simulink model "PVTOL_FE_and_FTC_Sim"  (R2021a)
settings: Solver=VariableStepAuto  StartTime=0.0  StopTime=10  RelTol=1e-3
values from neighbouring files (symbols this model uses):
  A_brevebar = [A_breve E_breve;zeros(2,4) zeros(2,2)]    [Quadcopter_Fault_Parameters_and_Flags.m]
  B_brevebar = [B_breve;zeros(2,2)]    [Quadcopter_Fault_Parameters_and_Flags.m]
  Delta_p = [1 1;1 -1]    [Quadcopter_Fault_Parameters_and_Flags.m]
  Delta_q = [1 1 1 1;1 -1 -1 1;1 1 -1 -1;-1 1 -1 1]    [Quadcopter_Fault_Parameters_and_Flags.m]
  g = 9.8066    [Quadcopter_Fault_Parameters_and_Flags.m]
  g_bar = [g_bold;zeros(2,1)]    [Quadcopter_Fault_Parameters_and_Flags.m]
  Jx = 0.0022    [Quadcopter_Fault_Parameters_and_Flags.m]
  K_D_kesi = diag([0.08,0.08,0.22])    [Quadcopter_Fault_Parameters_and_Flags.m]
  K_D_omega = diag([0.2,0.2,0.5])    [Quadcopter_Fault_Parameters_and_Flags.m]
  K_P_kesi = diag([0.18,0.18,052])    [Quadcopter_Fault_Parameters_and_Flags.m]
  K_P_omega = diag([1.5,1.5,2])    [Quadcopter_Fault_Parameters_and_Flags.m]
  kesi_d = [0 0 0]'    [Quadcopter_Fault_Parameters_and_Flags.m]
  kesi_dot_d = [0 0 0]'    [Quadcopter_Fault_Parameters_and_Flags.m]
  l = 0.1785    [Quadcopter_Fault_Parameters_and_Flags.m]
  Lf1 = 50    [Quadcopter_Fault_Parameters_and_Flags.m]
  Lf2 = 50    [Quadcopter_Fault_Parameters_and_Flags.m]
  LPI_brevebar = (P^-1)*M    [Quadcopter_Fault_Parameters_and_Flags.m]
  Ly1 = 0.009    [Quadcopter_Fault_Parameters_and_Flags.m]
  Ly2 = 5    [Quadcopter_Fault_Parameters_and_Flags.m]
  m = 0.4080    (= 0.408)    [Quadcopter_Fault_Parameters_and_Flags.m]
  O_d = [0 0 0]'    [Quadcopter_Fault_Parameters_and_Flags.m]
  Omega_d = [0 0 0]'    [Quadcopter_Fault_Parameters_and_Flags.m]
  Phi_dot_init = 0    [Quadcopter_Fault_Parameters_and_Flags.m]
  Phi_init = 0    [Quadcopter_Fault_Parameters_and_Flags.m]
  y_dot_init = 0    [Quadcopter_Fault_Parameters_and_Flags.m]
  y_init = 0    [Quadcopter_Fault_Parameters_and_Flags.m]
  z_dot_init = 0    [Quadcopter_Fault_Parameters_and_Flags.m]
  z_init = 0    [Quadcopter_Fault_Parameters_and_Flags.m]
settings Model: PauseTimes=2  Creator=kiankhaneghahi  LastModifiedBy=kiankhaneghahi

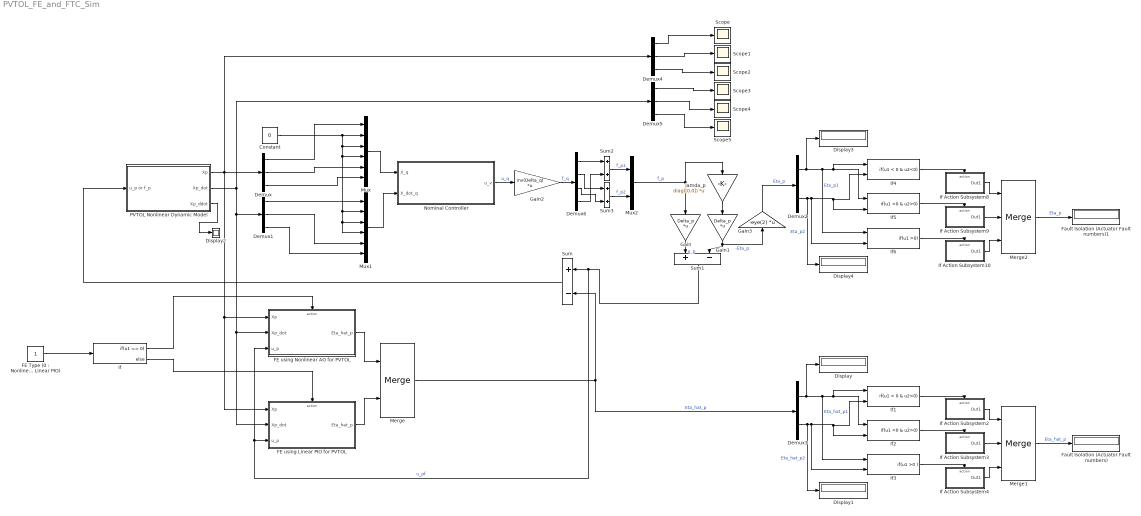
== system PVTOL_FE_and_FTC_Sim ==
  Constant : Constant  Value=0
  Demux{,1,4..5} (4 alike) : Demux  Outputs=3
  Demux2 : Demux  Outputs=2
  Demux3 : Demux  Outputs=2
  Demux6 : Demux
  Display{,1..4} (5 alike) : Display
  "FE Type (0 : Nonlinear AO - 1 : Linear PIO)" : Constant
  FE using Linear PIO for PVTOL : Subsystem
  FE using Nonlinear AO for PVTOL : Subsystem
  Fault Isolation (Actuator Fault numbers) : Display
  Fault Isolation (Actuator Fault numbers)1 : Display
  Gain : Gain  Gain=Delta_p  Multiplication=Matrix(K*u)
  Gain1 : Gain  Gain=Delta_p  Multiplication=Matrix(K*u)
  Gain2 : Gain  Gain=inv(Delta_q)  Multiplication=Matrix(K*u)
  Gain3 : Gain  Gain=-eye(2)  Multiplication=Matrix(K*u)
  If : If  IfExpression=u1 == 0
  If Action Subsystem10 : Subsystem  TreatAsAtomicUnit=on
  If Action Subsystem2 : Subsystem  TreatAsAtomicUnit=on
  If Action Subsystem3 : Subsystem  TreatAsAtomicUnit=on
  If Action Subsystem4 : Subsystem  TreatAsAtomicUnit=on
  If Action Subsystem8 : Subsystem  TreatAsAtomicUnit=on
  If Action Subsystem9 : Subsystem  TreatAsAtomicUnit=on
  If1 : If  NumInputs=2  IfExpression=u1 < 0 & u2<0  ShowElse=off
  If2 : If  NumInputs=2  IfExpression=u1 <0 & u2>0  ShowElse=off
  If3 : If  NumInputs=2  IfExpression=u1 >0  ShowElse=off
  If4 : If  NumInputs=2  IfExpression=u1 < 0 & u2<0  ShowElse=off
  If5 : If  NumInputs=2  IfExpression=u1 <0 & u2>0  ShowElse=off
  If6 : If  NumInputs=2  IfExpression=u1 >0  ShowElse=off
  Merge : Merge
  Merge1 : Merge  Inputs=3
  Merge2 : Merge  Inputs=3
  Mux : Mux  Inputs=6
  Mux1 : Mux  Inputs=6
  Mux2 : Mux  Inputs=2
  Nominal Controller : Subsystem
  PVTOL Nonlinear Dynamic Model : Subsystem
  Scope{,1..5} (6 alike) : Scope
  Sum : Sum  Inputs=+-
  Sum1 : Sum  Inputs=+-
  Sum2 : Sum
  Sum3 : Sum
  lamda_p : Gain  Gain=diag([0,0])  Multiplication=Matrix(K*u)
  wires:
  PVTOL Nonlinear Dynamic Model/1(Xp) -> Demux4/1, FE using Linear PIO for PVTOL/1(Xp), FE using Nonlinear AO for PVTOL/1(Xp), Demux/1
  PVTOL Nonlinear Dynamic Model/2(Xp_dot) -> Demux5/1, FE using Linear PIO for PVTOL/2(Xp_dot), FE using Nonlinear AO for PVTOL/2(Xp_dot), Demux1/1
  Mux/1 -> Nominal Controller/1(X_q)
  Demux/1 -> Mux/1
  Demux/2 -> Mux/5
  Demux/3 -> Mux/6
  Mux1/1 -> Nominal Controller/2(X_dot_q)
  Demux1/1 -> Mux1/1
  Demux1/2 -> Mux1/5
  Demux1/3 -> Mux1/6
  Constant/1 -> Mux1/4, Mux1/3, Mux1/2, Mux/4, Mux/3, Mux/2
  "FE Type (0 : Nonlinear AO - 1 : Linear PIO)"/1 -> If/1
  If/1 -> FE using Nonlinear AO for PVTOL/Action
  If/2 -> FE using Linear PIO for PVTOL/Action
  FE using Nonlinear AO for PVTOL/1(Eta_hat_p) -> Merge/1
  FE using Linear PIO for PVTOL/1(Eta_hat_p) -> Merge/2
  Sum1/1 -> FE using Linear PIO for PVTOL/3(u_p), FE using Nonlinear AO for PVTOL/3(u_p), Sum/1  "u_pf"
  Merge/1 -> Demux3/1, Sum/2  "Eta_hat_p"
  Sum/1 -> PVTOL Nonlinear Dynamic Model/1(u_p or f_p)
  If Action Subsystem4/1(Out1) -> Merge1/3
  Merge1/1 -> Fault Isolation (Actuator Fault numbers)/1  "Eta_hat_p"
  If1/1 -> If Action Subsystem2/Action
  Demux3/1 -> Display/1, If3/1, If1/1, If2/1  "Eta_hat_p1"
  If Action Subsystem3/1(Out1) -> Merge1/2
  Demux3/2 -> Display1/1, If3/2, If1/2, If2/2  "Eta_hat_p2"
  If Action Subsystem2/1(Out1) -> Merge1/1
  If3/1 -> If Action Subsystem4/Action
  If2/1 -> If Action Subsystem3/Action
  PVTOL Nonlinear Dynamic Model/3(Xp_ddot) -> Display2/1
  Demux4/1 -> Scope/1
  Demux4/2 -> Scope1/1
  Demux4/3 -> Scope2/1
  Demux5/1 -> Scope3/1
  Demux5/2 -> Scope4/1
  Demux5/3 -> Scope5/1
  Gain2/1 -> Demux6/1  "f_q"
  Gain/1 -> Sum1/1  "u_p"
  Gain1/1 -> Sum1/2, Gain3/1  "-Eta_p"
  lamda_p/1 -> Gain1/1
  Nominal Controller/1(u_v) -> Gain2/1  "u_q"
  Demux6/1 -> Sum2/1
  Demux6/4 -> Sum2/2
  Demux6/2 -> Sum3/1
  Demux6/3 -> Sum3/2
  Sum2/1 -> Mux2/1  "f_p1"
  Sum3/1 -> Mux2/2  "f_p2"
  Mux2/1 -> Gain/1, lamda_p/1  "f_p"
  Gain3/1 -> Demux2/1  "Eta_p"
  Merge2/1 -> Fault Isolation (Actuator Fault numbers)1/1  "Eta_p"
  Demux2/1 -> Display3/1, If6/1, If4/1, If5/1  "Eta_p1"
  If6/1 -> If Action Subsystem10/Action
  If4/1 -> If Action Subsystem8/Action
  If5/1 -> If Action Subsystem9/Action
  Demux2/2 -> Display4/1, If6/2, If4/2, If5/2  "Eta_p2"
  If Action Subsystem8/1(Out1) -> Merge2/1
  If Action Subsystem9/1(Out1) -> Merge2/2
  If Action Subsystem10/1(Out1) -> Merge2/3

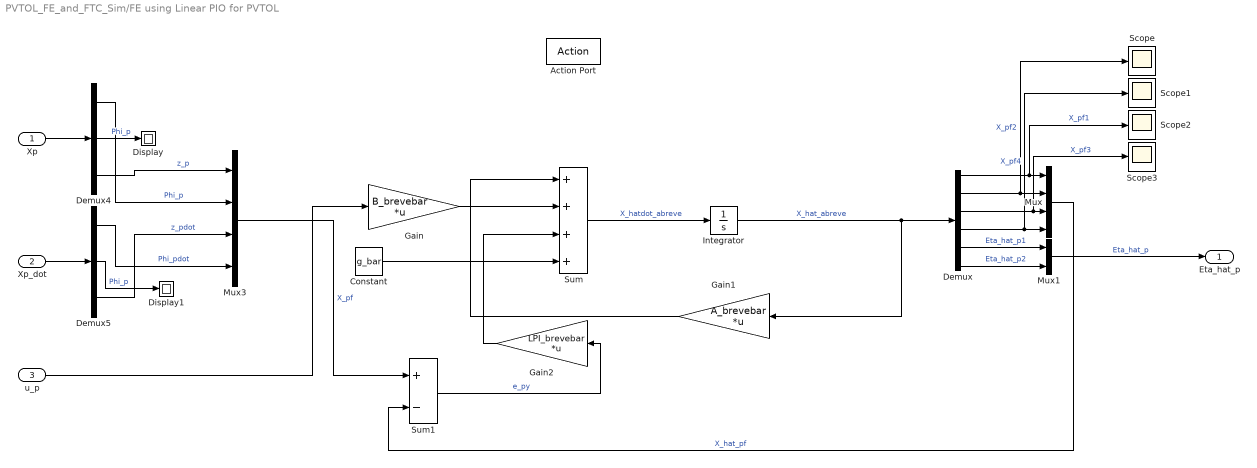
== system PVTOL_FE_and_FTC_Sim/FE using Linear PIO for PVTOL ==
  Xp : Inport
  Xp_dot : Inport  Port=2
  u_p : Inport  Port=3
  Action Port : ActionPort  ActionPortLabel=else
  Constant : Constant  Value=g_bar
  Demux : Demux  Outputs=6
  Demux4 : Demux  Outputs=3
  Demux5 : Demux  Outputs=3
  Display : Display
  Display1 : Display
  Gain : Gain  Gain=B_brevebar  Multiplication=Matrix(K*u)
  Gain1 : Gain  Gain=A_brevebar  Multiplication=Matrix(K*u)
  Gain2 : Gain  Gain=LPI_brevebar  Multiplication=Matrix(K*u)
  Integrator : Integrator
  Mux : Mux
  Mux1 : Mux  Inputs=2
  Mux3 : Mux
  Scope{,1..3} (4 alike) : Scope
  Sum : Sum  Inputs=++++
  Sum1 : Sum  Inputs=+-
  Eta_hat_p : Outport
  wires:
  Demux5/1 -> Mux3/4  "Phi_pdot"
  Xp/1 -> Demux4/1
  u_p/1 -> Gain/1
  Demux4/1 -> Mux3/2  "Phi_p"
  Demux4/3 -> Mux3/1  "z_p"
  Demux5/3 -> Mux3/3  "z_pdot"
  Xp_dot/1 -> Demux5/1
  Mux1/1 -> Eta_hat_p/1  "Eta_hat_p"
  Integrator/1 -> Demux/1, Gain1/1  "X_hat_abreve"
  Sum/1 -> Integrator/1  "X_hatdot_abreve"
  Gain1/1 -> Sum/1
  Gain/1 -> Sum/2
  Constant/1 -> Sum/4
  Demux/6 -> Mux1/2  "Eta_hat_p2"
  Demux/5 -> Mux1/1  "Eta_hat_p1"
  Mux/1 -> Sum1/2  "X_hat_pf"
  Demux4/2 -> Display/1  "Phi_p"
  Demux5/2 -> Display1/1  "Phi_p"
  Mux3/1 -> Sum1/1  "X_pf"
  Gain2/1 -> Sum/3
  Sum1/1 -> Gain2/1  "e_py"
  Demux/2 -> Scope/1, Mux/2  "X_pf2"
  Demux/3 -> Scope3/1, Mux/3  "X_pf3"
  Demux/1 -> Scope2/1, Mux/1  "X_pf1"
  Demux/4 -> Scope1/1, Mux/4  "X_pf4"

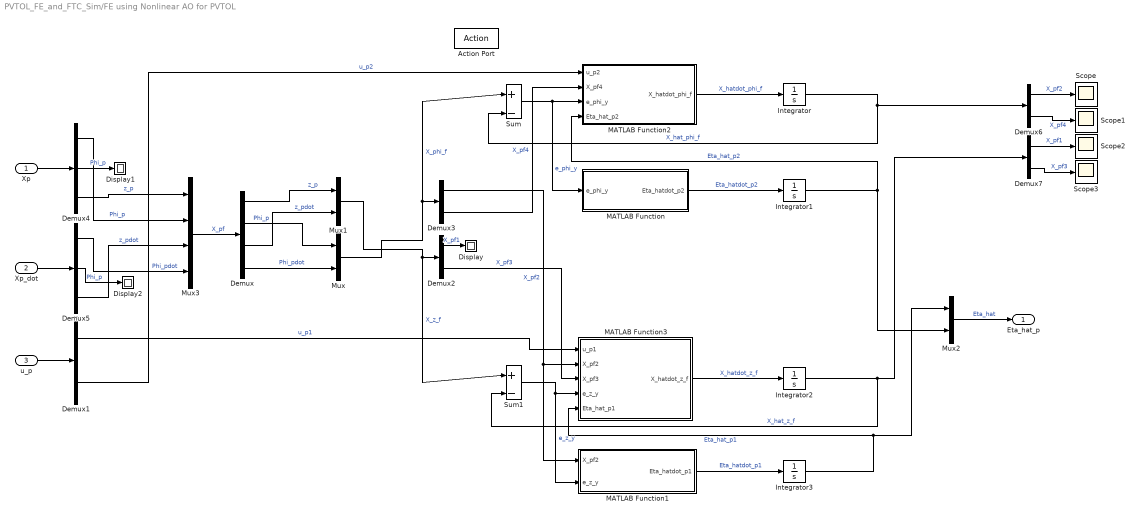
== system PVTOL_FE_and_FTC_Sim/FE using Nonlinear AO for PVTOL ==
  Xp : Inport
  Xp_dot : Inport  Port=2
  u_p : Inport  Port=3
  Action Port : ActionPort  ActionPortLabel=if(u1 == 0)
  Demux : Demux
  Demux{1..3,6..7} (5 alike) : Demux  Outputs=2
  Demux4 : Demux  Outputs=3
  Demux5 : Demux  Outputs=3
  Display : Display
  Display1 : Display
  Display2 : Display
  Integrator{,1..3} (4 alike) : Integrator
  MATLAB Function : MATLAB Function  TreatAsAtomicUnit=on
  MATLAB Function1 : MATLAB Function  TreatAsAtomicUnit=on
  MATLAB Function2 : MATLAB Function  TreatAsAtomicUnit=on
  MATLAB Function3 : MATLAB Function  TreatAsAtomicUnit=on
  Mux : Mux  Inputs=2
  Mux1 : Mux  Inputs=2
  Mux2 : Mux  Inputs=2
  Mux3 : Mux
  Scope{,1..3} (4 alike) : Scope
  Sum : Sum  Inputs=|+-
  Sum1 : Sum  Inputs=|+-
  Eta_hat_p : Outport
  wires:
  MATLAB Function3/1(X_hatdot_z_f) -> Integrator2/1  "X_hatdot_z_f"
  MATLAB Function2/1(X_hatdot_phi_f) -> Integrator/1  "X_hatdot_phi_f"
  Demux/2 -> Mux/1  "Phi_p"
  Demux/4 -> Mux/2  "Phi_pdot"
  Demux/3 -> Mux1/2  "z_pdot"
  Demux/1 -> Mux1/1  "z_p"
  Mux/1 -> Demux3/1, Sum/1  "X_phi_f"
  u_p/1 -> Demux1/1
  MATLAB Function1/1(Eta_hatdot_p1) -> Integrator3/1  "Eta_hatdot_p1"
  MATLAB Function/1(Eta_hatdot_p2) -> Integrator1/1  "Eta_hatdot_p2"
  Sum/1 -> MATLAB Function/1(e_phi_y), MATLAB Function2/3(e_phi_y)  "e_phi_y"
  Sum1/1 -> MATLAB Function1/2(e_z_y), MATLAB Function3/4(e_z_y)  "e_z_y"
  Mux1/1 -> Sum1/1, Demux2/1  "X_z_f"
  Demux2/2 -> MATLAB Function3/3(X_pf3)  "X_pf3"
  Demux3/2 -> MATLAB Function2/2(X_pf4)  "X_pf4"
  Demux3/1 -> MATLAB Function3/2(X_pf2), MATLAB Function1/1(X_pf2)  "X_pf2"
  Demux1/1 -> MATLAB Function3/1(u_p1)  "u_p1"
  Demux1/2 -> MATLAB Function2/1(u_p2)  "u_p2"
  Integrator1/1 -> Mux2/2, MATLAB Function2/4(Eta_hat_p2)  "Eta_hat_p2"
  Integrator3/1 -> Mux2/1, MATLAB Function3/5(Eta_hat_p1)  "Eta_hat_p1"
  Mux2/1 -> Eta_hat_p/1  "Eta_hat"
  Xp/1 -> Demux4/1
  Mux3/1 -> Demux/1  "X_pf"
  Xp_dot/1 -> Demux5/1
  Demux4/3 -> Mux3/1  "z_p"
  Demux5/3 -> Mux3/3  "z_pdot"
  Demux4/1 -> Mux3/2  "Phi_p"
  Demux5/1 -> Mux3/4  "Phi_pdot"
  Demux2/1 -> Display/1  "X_pf1"
  Demux4/2 -> Display1/1  "Phi_p"
  Demux5/2 -> Display2/1  "Phi_p"
  Integrator/1 -> Sum/2, Demux6/1  "X_hat_phi_f"
  Integrator2/1 -> Demux7/1, Sum1/2  "X_hat_z_f"
  Demux7/2 -> Scope3/1  "X_pf3"
  Demux7/1 -> Scope2/1  "X_pf1"
  Demux6/1 -> Scope/1  "X_pf2"
  Demux6/2 -> Scope1/1  "X_pf4"

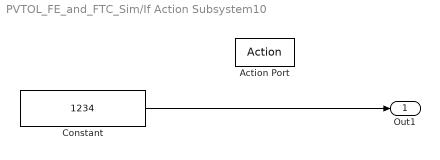
== system PVTOL_FE_and_FTC_Sim/If Action Subsystem10 ==
  Action Port : ActionPort  ActionPortLabel=if(u1 >0)
  Constant : Constant  Value=1234
  Out1 : Outport
  wires:
  Constant/1 -> Out1/1

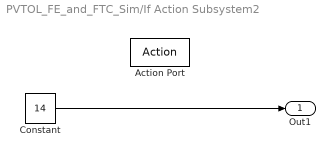
== system PVTOL_FE_and_FTC_Sim/If Action Subsystem2 ==
  Action Port : ActionPort  ActionPortLabel=if(u1 < 0 & u2<0)
  Constant : Constant  Value=14
  Out1 : Outport
  wires:
  Constant/1 -> Out1/1

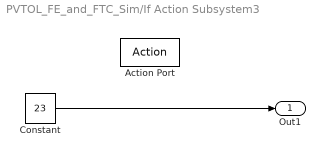
== system PVTOL_FE_and_FTC_Sim/If Action Subsystem3 ==
  Action Port : ActionPort  ActionPortLabel=if(u1 <0 & u2>0)
  Constant : Constant  Value=23
  Out1 : Outport
  wires:
  Constant/1 -> Out1/1

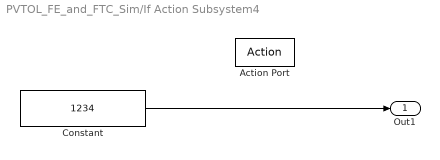
== system PVTOL_FE_and_FTC_Sim/If Action Subsystem4 ==
  Action Port : ActionPort  ActionPortLabel=if(u1 >0 )
  Constant : Constant  Value=1234
  Out1 : Outport
  wires:
  Constant/1 -> Out1/1

== system PVTOL_FE_and_FTC_Sim/If Action Subsystem8 ==
  Action Port : ActionPort  ActionPortLabel=if(u1 < 0 & u2<0)
  Constant : Constant  Value=14
  Out1 : Outport
  wires:
  Constant/1 -> Out1/1

== system PVTOL_FE_and_FTC_Sim/If Action Subsystem9 ==
  Action Port : ActionPort  ActionPortLabel=if(u1 <0 & u2>0)
  Constant : Constant  Value=23
  Out1 : Outport
  wires:
  Constant/1 -> Out1/1

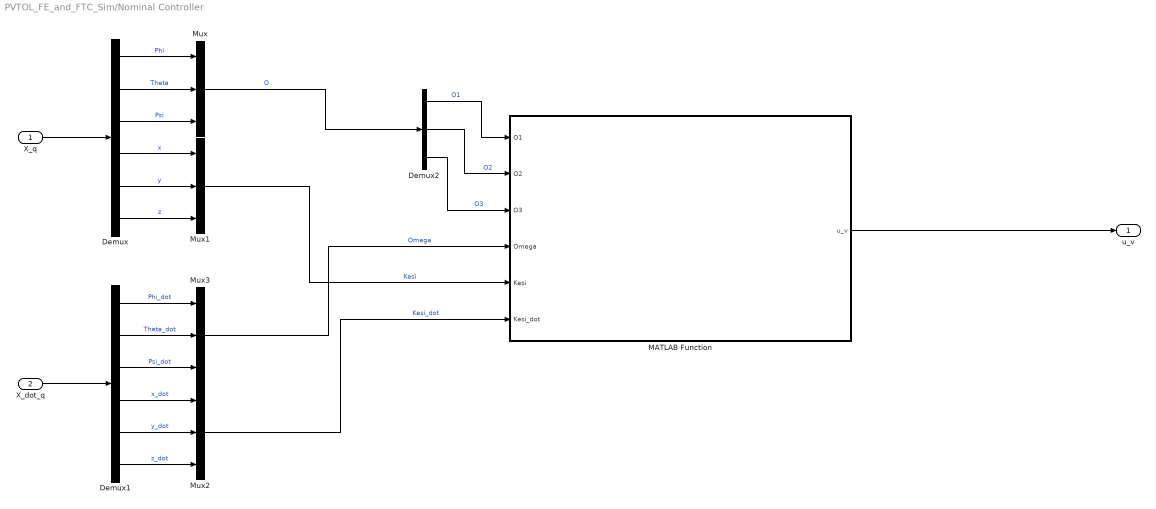
== system PVTOL_FE_and_FTC_Sim/Nominal Controller ==
  X_q : Inport
  X_dot_q : Inport  Port=2
  Demux : Demux  Outputs=6
  Demux1 : Demux  Outputs=6
  Demux2 : Demux  Outputs=3
  MATLAB Function : MATLAB Function  TreatAsAtomicUnit=on
  Mux{,1..3} (4 alike) : Mux  Inputs=3
  u_v : Outport
  wires:
  X_q/1 -> Demux/1
  X_dot_q/1 -> Demux1/1
  Demux/3 -> Mux/3  "Psi"
  Demux/2 -> Mux/2  "Theta"
  Demux/1 -> Mux/1  "Phi"
  Demux/4 -> Mux1/1  "x"
  Demux/5 -> Mux1/2  "y"
  Demux/6 -> Mux1/3  "z"
  Demux1/4 -> Mux2/1  "x_dot"
  Demux1/5 -> Mux2/2  "y_dot"
  Demux1/6 -> Mux2/3  "z_dot"
  MATLAB Function/1(u_v) -> u_v/1
  Demux1/1 -> Mux3/1  "Phi_dot"
  Demux1/2 -> Mux3/2  "Theta_dot"
  Demux1/3 -> Mux3/3  "Psi_dot"
  Mux1/1 -> MATLAB Function/5(Kesi)  "Kesi"
  Mux2/1 -> MATLAB Function/6(Kesi_dot)  "Kesi_dot"
  Mux/1 -> Demux2/1  "O"
  Demux2/1 -> MATLAB Function/1(O1)  "O1"
  Demux2/2 -> MATLAB Function/2(O2)  "O2"
  Demux2/3 -> MATLAB Function/3(O3)  "O3"
  Mux3/1 -> MATLAB Function/4(Omega)  "Omega"

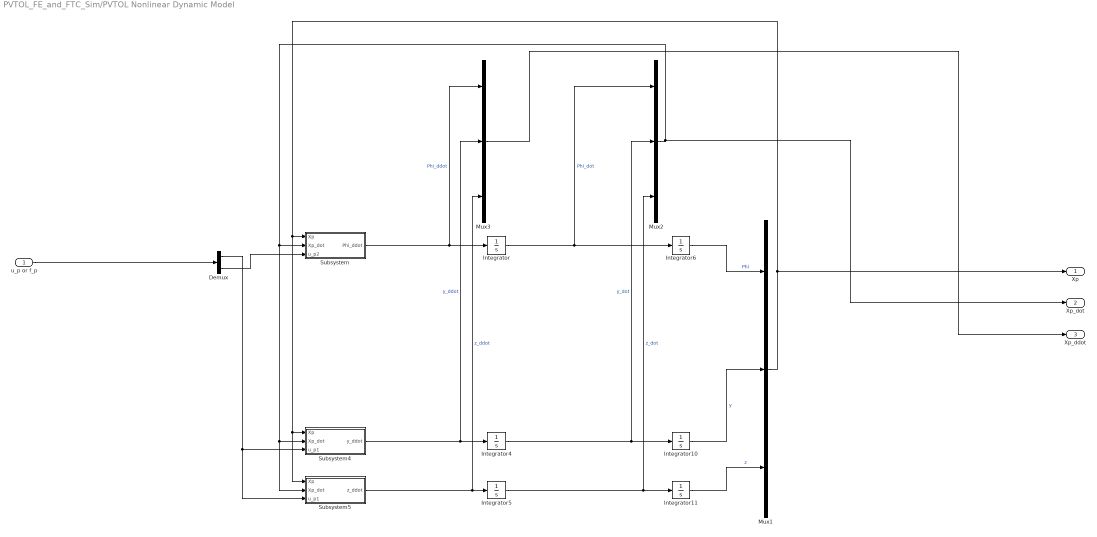
== system PVTOL_FE_and_FTC_Sim/PVTOL Nonlinear Dynamic Model ==
  u_p or f_p : Inport
  Demux : Demux  Outputs=2
  Integrator : Integrator  InitialCondition=Phi_dot_init
  Integrator10 : Integrator  InitialCondition=y_init
  Integrator11 : Integrator  InitialCondition=z_init
  Integrator4 : Integrator  InitialCondition=y_dot_init
  Integrator5 : Integrator  InitialCondition=z_dot_init
  Integrator6 : Integrator  InitialCondition=Phi_init
  Mux1 : Mux  Inputs=3
  Mux2 : Mux  Inputs=3
  Mux3 : Mux  Inputs=3
  Subsystem : Subsystem
  Subsystem4 : Subsystem
  Subsystem5 : Subsystem
  Xp : Outport
  Xp_dot : Outport  Port=2
  Xp_ddot : Outport  Port=3
  wires:
  Integrator/1 -> Integrator6/1, Mux2/1  "Phi_dot"
  Integrator4/1 -> Mux2/2, Integrator10/1  "y_dot"
  Integrator5/1 -> Mux2/3, Integrator11/1  "z_dot"
  Subsystem/1(Phi_ddot) -> Mux3/1, Integrator/1  "Phi_ddot"
  Subsystem5/1(z_ddot) -> Mux3/3, Integrator5/1  "z_ddot"
  Subsystem4/1(y_ddot) -> Integrator4/1, Mux3/2  "y_ddot"
  u_p or f_p/1 -> Demux/1
  Demux/2 -> Subsystem/3(u_p2)
  Demux/1 -> Subsystem5/3(u_p1), Subsystem4/3(u_p1)
  Integrator6/1 -> Mux1/1  "Phi"
  Integrator10/1 -> Mux1/2  "y"
  Integrator11/1 -> Mux1/3  "z"
  Mux1/1 -> Xp/1, Subsystem5/1(Xp), Subsystem4/1(Xp), Subsystem/1(Xp)
  Mux2/1 -> Xp_dot/1, Subsystem5/2(Xp_dot), Subsystem4/2(Xp_dot), Subsystem/2(Xp_dot)
  Mux3/1 -> Xp_ddot/1

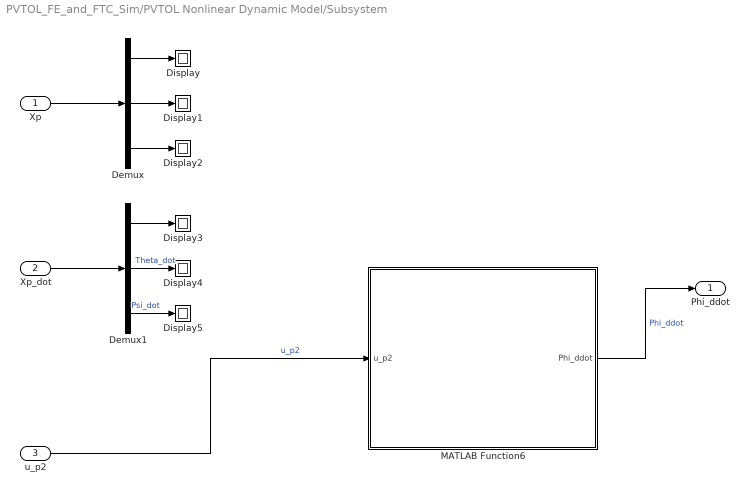
== system PVTOL_FE_and_FTC_Sim/PVTOL Nonlinear Dynamic Model/Subsystem ==
  Xp : Inport
  Xp_dot : Inport  Port=2
  u_p2 : Inport  Port=3
  Demux : Demux  Outputs=3
  Demux1 : Demux  Outputs=3
  Display{,1..5} (6 alike) : Display
  MATLAB Function6 : MATLAB Function  TreatAsAtomicUnit=on
  Phi_ddot : Outport
  wires:
  Xp/1 -> Demux/1
  Xp_dot/1 -> Demux1/1
  u_p2/1 -> MATLAB Function6/1(u_p2)  "u_p2"
  MATLAB Function6/1(Phi_ddot) -> Phi_ddot/1  "Phi_ddot"
  Demux/1 -> Display/1
  Demux/2 -> Display1/1
  Demux/3 -> Display2/1
  Demux1/1 -> Display3/1
  Demux1/2 -> Display4/1  "Theta_dot"
  Demux1/3 -> Display5/1  "Psi_dot"

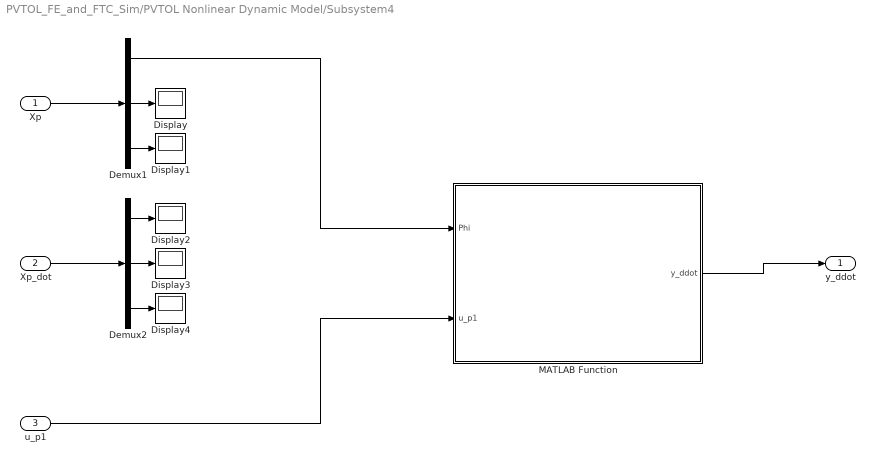
== system PVTOL_FE_and_FTC_Sim/PVTOL Nonlinear Dynamic Model/Subsystem4 ==
  Xp : Inport
  Xp_dot : Inport  Port=2
  u_p1 : Inport  Port=3
  Demux1 : Demux  Outputs=3
  Demux2 : Demux  Outputs=3
  Display{,1..4} (5 alike) : Display
  MATLAB Function : MATLAB Function  TreatAsAtomicUnit=on
  y_ddot : Outport
  wires:
  MATLAB Function/1(y_ddot) -> y_ddot/1
  Xp_dot/1 -> Demux2/1
  Xp/1 -> Demux1/1
  u_p1/1 -> MATLAB Function/2(u_p1)
  Demux1/1 -> MATLAB Function/1(Phi)
  Demux1/2 -> Display/1
  Demux1/3 -> Display1/1
  Demux2/1 -> Display2/1
  Demux2/2 -> Display3/1
  Demux2/3 -> Display4/1

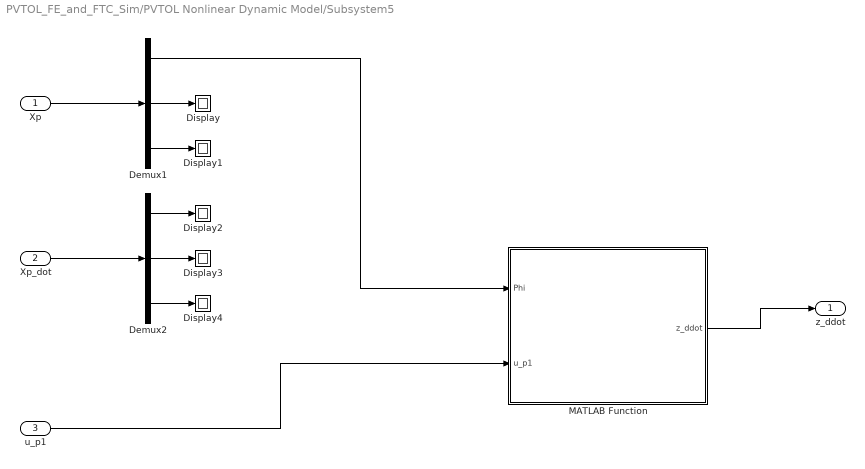
== system PVTOL_FE_and_FTC_Sim/PVTOL Nonlinear Dynamic Model/Subsystem5 ==
  Xp : Inport
  Xp_dot : Inport  Port=2
  u_p1 : Inport  Port=3
  Demux1 : Demux  Outputs=3
  Demux2 : Demux  Outputs=3
  Display{,1..4} (5 alike) : Display
  MATLAB Function : MATLAB Function  TreatAsAtomicUnit=on
  z_ddot : Outport
  wires:
  Xp/1 -> Demux1/1
  Xp_dot/1 -> Demux2/1
  MATLAB Function/1(z_ddot) -> z_ddot/1
  u_p1/1 -> MATLAB Function/2(u_p1)
  Demux1/1 -> MATLAB Function/1(Phi)
  Demux1/2 -> Display/1
  Demux1/3 -> Display1/1
  Demux2/1 -> Display2/1
  Demux2/2 -> Display3/1
  Demux2/3 -> Display4/1

== matlab function PVTOL_FE_and_FTC_Sim/PVTOL Nonlinear Dynamic Model/Subsystem/MATLAB Function6 ==
  data: u_p2 input; Phi_ddot output; l parameter; Jx parameter
function Phi_ddot = fcn(u_p2, l, Jx)

Phi_ddot = (l/Jx)*u_p2;

== matlab function PVTOL_FE_and_FTC_Sim/FE using Nonlinear AO for PVTOL/MATLAB Function ==
  data: e_phi_y input; Eta_hatdot_p2 output; l parameter; Jx parameter; Lf1 parameter
function Eta_hatdot_p2 = fcn(e_phi_y, l, Jx, Lf1)
beta1 = [0;l/Jx];
Eta_hatdot_p2 = -Lf1*(beta1')*e_phi_y;

== matlab function PVTOL_FE_and_FTC_Sim/FE using Nonlinear AO for PVTOL/MATLAB Function1 ==
  data: X_pf2 input; e_z_y input; Eta_hatdot_p1 output; m parameter; Lf2 parameter
function Eta_hatdot_p1 = fcn(X_pf2, e_z_y, m, Lf2)
beta2 = [0;cos(X_pf2)/m];
Eta_hatdot_p1 = -Lf2*(beta2')*e_z_y;

== matlab function PVTOL_FE_and_FTC_Sim/FE using Nonlinear AO for PVTOL/MATLAB Function2 ==
  data: u_p2 input; X_pf4 input; e_phi_y input; X_hatdot_phi_f output; Eta_hat_p2 input; l parameter; Jx parameter; Ly1 parameter
function X_hatdot_phi_f = fcn(u_p2, X_pf4, e_phi_y, Eta_hat_p2, l, Jx, Ly1)
alpha1 = [X_pf4;l*u_p2/Jx];
beta1 = [0;l/Jx];
X_hatdot_phi_f = alpha1 + beta1*Eta_hat_p2 - Ly1*e_phi_y;

== matlab function PVTOL_FE_and_FTC_Sim/PVTOL Nonlinear Dynamic Model/Subsystem4/MATLAB Function ==
  data: Phi input; u_p1 input; y_ddot output; m parameter
function y_ddot = fcn(Phi,u_p1, m)

y_ddot = -sin(Phi)*(1/m)*u_p1;

== matlab function PVTOL_FE_and_FTC_Sim/PVTOL Nonlinear Dynamic Model/Subsystem5/MATLAB Function ==
  data: Phi input; u_p1 input; z_ddot output; g parameter; m parameter
function z_ddot = fcn(Phi, u_p1, g, m)

z_ddot = -g + cos(Phi)*(1/m)*u_p1;

== matlab function PVTOL_FE_and_FTC_Sim/FE using Nonlinear AO for PVTOL/MATLAB Function3 ==
  data: u_p1 input; X_pf2 input; X_pf3 input; e_z_y input; X_hatdot_z_f output; Eta_hat_p1 input; m parameter; g parameter; Ly2 parameter
function X_hatdot_z_f = fcn(u_p1, X_pf2, X_pf3, e_z_y, Eta_hat_p1, m, g, Ly2)
alpha2 = [X_pf3;(cos(X_pf2)*u_p1/m)-g];
beta2 = [0;cos(X_pf2)/m];
X_hatdot_z_f = alpha2 + beta2*Eta_hat_p1 - Ly2*e_z_y;

== matlab function PVTOL_FE_and_FTC_Sim/Nominal Controller/MATLAB Function ==
  data: O1 input; O2 input; O3 input; Omega input; u_v output; Kesi input; Kesi_dot input; K_P_kesi parameter; kesi_d parameter; K_D_kesi parameter; kesi_dot_d parameter; K_P_omega parameter; K_D_omega parameter; Omega_d parameter; O_d parameter
function u_v = fcn(O1, O2, O3, Omega, Kesi, Kesi_dot, K_P_kesi, kesi_d, K_D_kesi, kesi_dot_d, K_P_omega, K_D_omega, Omega_d, O_d)
O = [O1,O2,O3]';
q = quaternion(O','euler','xyz','frame');
q_d = quaternion(O_d','euler','xyz','frame');
q_d_conj = conj(q_d);
q_e = q * q_d_conj;
%q_e_ln = 2*log(q_e);
q_e_eu = euler(q_e,'xyz','frame')';
u_v = [norm(-K_P_kesi*(Kesi-kesi_d)-K_D_kesi*(Kesi_dot-kesi_dot_d));-K_P_omega*q_e_eu-K_D_omega*(Omega-Omega_d)];
